simulink model "lab7"  (R2012b)
settings: Solver=ode45  StartTime=0.0  StopTime=720  RelTol=1e-3
undefined symbols (not defined in the file): des, gcbh
settings Model: Creator=gick  LastModifiedBy=gick

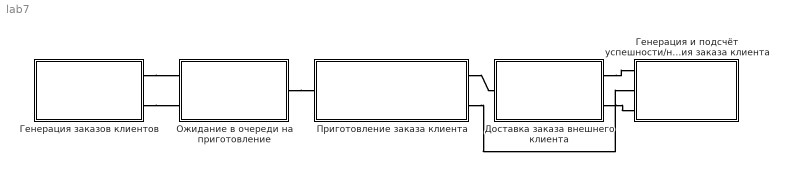
== system lab7 ==
  Генерация заказов клиентов : Subsystem
  Генерация и подсчёт успешности/неуспешности выполнения заказа клиента : Subsystem
  Доставка заказа внешнего клиента : Subsystem
  Ожидание в очереди на приготовление : Subsystem
  Приготовление заказа клиента : Subsystem
  connections:
  Генерация заказов клиентов/RConn1 -- Ожидание в очереди на приготовление/LConn1
  Генерация заказов клиентов/RConn2 -- Ожидание в очереди на приготовление/LConn2
  Ожидание в очереди на приготовление/RConn1 -- Приготовление заказа клиента/LConn1
  Приготовление заказа клиента/RConn1 -- Доставка заказа внешнего клиента/LConn1
  Приготовление заказа клиента/RConn2 -- Генерация и подсчёт успешности/неуспешности выполнения заказа клиента/LConn2
  Доставка заказа внешнего клиента/RConn1 -- Генерация и подсчёт успешности/неуспешности выполнения заказа клиента/LConn1
  Доставка заказа внешнего клиента/RConn2 -- Генерация и подсчёт успешности/неуспешности выполнения заказа клиента/LConn3

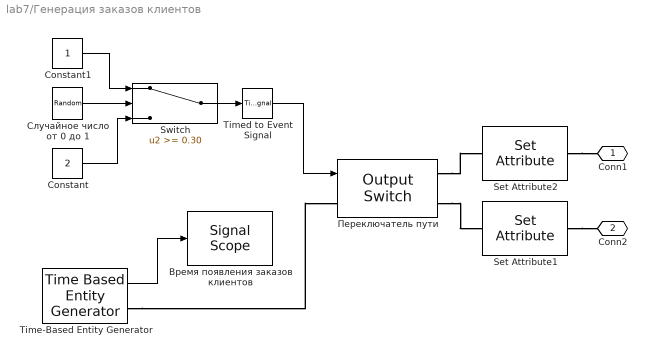
== system lab7/Генерация заказов клиентов ==
  Constant : Constant  Value=2
  Constant1 : Constant
  Set Attribute1 : SetAttribute  AttributeName=client_type  AttributeValue=2  EvaluatedAttributeValue={ 2 }
  Set Attribute2 : SetAttribute  AttributeName=client_type  EvaluatedAttributeValue={ 1 }
  Switch : Switch  Threshold=0.30
  Time-Based Entity Generator : TimeBasedEntityGenerator  Distribution=Exponential  InitialSeed=12  Mean=15  PriorityEntityGeneration=500  StatAverageIntergenerationTime=on
      settings: OutputPortMap=o2
  Timed to Event Signal : TimedToEventSignal
  Время появления заказов клиентов : SignalScope  LoadFcn=des.scope.CallbackSupport('seLoadFcn',gcbh)  StartFcn=des.scope.CallbackSupport('seStartFcn',gcbh)  StopFcn=des.scope.CallbackSupport('seStopFcn',gcbh)  ShowCountPlotted=on
      settings: CopyFcn=des.scope.CallbackSupport('seCopyFcn',gcbh)  DeleteFcn=des.scope.CallbackSupport('seDeleteFcn',gcbh)  PreSaveFcn=des.scope.CallbackSupport('sePreSaveFcn',gcbh)  NameChangeFcn=des.scope.CallbackSupport('seNameChangeFcn',gcbh)  OpenFcn=des.scope.CallbackSupport('seOpenFcn',gcbh)
  "Переключатель пути " : OutputSwitch  NumberOutputPorts=2  SwitchingCriterion=From signal port p
  Случайное число от 0 до 1 : UniformRandomNumber  Minimum=0  Seed=12  SampleTime=0.1
  Conn1 : PMIOPort  Port=1  Side=Right
  Conn2 : PMIOPort  Port=2  Side=Right
  wires:
  Случайное число от 0 до 1/1 -> Switch/2
  Switch/1 -> Timed to Event Signal/1
  Timed to Event Signal/1 -> "Переключатель пути "/1
  Time-Based Entity Generator/1 -> Время появления заказов клиентов/1
  Constant/1 -> Switch/3
  Constant1/1 -> Switch/1
  connections:
  Time-Based Entity Generator/RConn1 -- "Переключатель пути "/LConn1
  Set Attribute1/RConn1 -- Conn2/RConn1
  Set Attribute2/RConn1 -- Conn1/RConn1
  "Переключатель пути "/RConn1 -- Set Attribute2/LConn1
  "Переключатель пути "/RConn2 -- Set Attribute1/LConn1

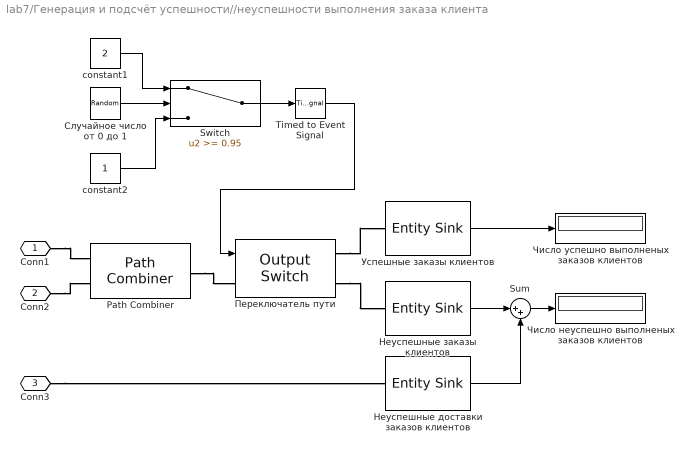
== system lab7/Генерация и подсчёт успешности//неуспешности выполнения заказа клиента ==
  Path Combiner : PathCombiner  NumberInputPorts=2
  Sum : Sum  Inputs=|++
  Switch : Switch  Threshold=0.95
  Timed to Event Signal : TimedToEventSignal
  constant1 : Constant  Value=2
  constant2 : Constant
  Неуспешные доставки заказов клиентов : EntitySink  StatNumberArrived=on
  Неуспешные заказы клиентов : EntitySink  StatNumberArrived=on
  "Переключатель пути " : OutputSwitch  NumberOutputPorts=2  SwitchingCriterion=From signal port p
  Случайное число от 0 до 1 : UniformRandomNumber  Minimum=0  Seed=12  SampleTime=0.1
  Успешные заказы клиентов : EntitySink  StatNumberArrived=on
  Число неуспешно выполненых заказов клиентов : Display
  Число успешно выполненых заказов клиентов : Display
  Conn1 : PMIOPort  Port=1  Side=Left
  Conn2 : PMIOPort  Port=2  Side=Left
  Conn3 : PMIOPort  Port=3  Side=Left
  wires:
  constant1/1 -> Switch/1
  constant2/1 -> Switch/3
  Случайное число от 0 до 1/1 -> Switch/2
  Switch/1 -> Timed to Event Signal/1
  Timed to Event Signal/1 -> "Переключатель пути "/1
  Успешные заказы клиентов/1 -> Число успешно выполненых заказов клиентов/1
  Неуспешные доставки заказов клиентов/1 -> Sum/2
  Неуспешные заказы клиентов/1 -> Sum/1
  Sum/1 -> Число неуспешно выполненых заказов клиентов/1
  connections:
  Path Combiner/RConn1 -- "Переключатель пути "/LConn1
  Conn1/RConn1 -- Path Combiner/LConn1
  Conn2/RConn1 -- Path Combiner/LConn2
  "Переключатель пути "/RConn1 -- Успешные заказы клиентов/LConn1
  "Переключатель пути "/RConn2 -- Неуспешные заказы клиентов/LConn1
  Conn3/RConn1 -- Неуспешные доставки заказов клиентов/LConn1

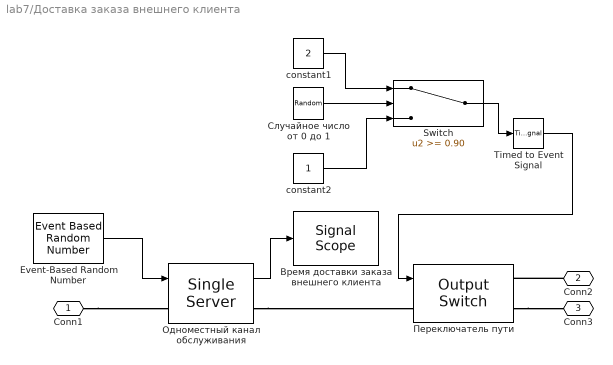
== system lab7/Доставка заказа внешнего клиента ==
  Event-Based Random Number : EventBasedRandomNumber  Distribution=Uniform  minUnif=10  maxUnif=50  Seed=12
  Switch : Switch  Threshold=0.90
  Timed to Event Signal : TimedToEventSignal
  constant1 : Constant  Value=2
  constant2 : Constant
  Время доставки заказа внешнего клиента : SignalScope  LoadFcn=des.scope.CallbackSupport('seLoadFcn',gcbh)  StartFcn=des.scope.CallbackSupport('seStartFcn',gcbh)  StopFcn=des.scope.CallbackSupport('seStopFcn',gcbh)  XMax=640  ShowCountPlotted=on
      settings: CopyFcn=des.scope.CallbackSupport('seCopyFcn',gcbh)  DeleteFcn=des.scope.CallbackSupport('seDeleteFcn',gcbh)  PreSaveFcn=des.scope.CallbackSupport('sePreSaveFcn',gcbh)  NameChangeFcn=des.scope.CallbackSupport('seNameChangeFcn',gcbh)  OpenFcn=des.scope.CallbackSupport('seOpenFcn',gcbh)  YMax=20
  Одноместный канал обслуживания : SingleServer  ServiceTimeFrom=Signal port t  AttributeName=ServTime  StatAverageWait=on
      settings: OutputPortMap=o4
  "Переключатель пути " : OutputSwitch  NumberOutputPorts=2  SwitchingCriterion=From signal port p
  Случайное число от 0 до 1 : UniformRandomNumber  Minimum=0  Seed=12  SampleTime=0.1
  Conn1 : PMIOPort  Port=1  Side=Left
  Conn2 : PMIOPort  Port=2  Side=Right
  Conn3 : PMIOPort  Port=3  Side=Right
  wires:
  Event-Based Random Number/1 -> Одноместный канал обслуживания/1
  Одноместный канал обслуживания/1 -> Время доставки заказа внешнего клиента/1
  constant1/1 -> Switch/1
  constant2/1 -> Switch/3
  Случайное число от 0 до 1/1 -> Switch/2
  Switch/1 -> Timed to Event Signal/1
  Timed to Event Signal/1 -> "Переключатель пути "/1
  connections:
  Conn1/RConn1 -- Одноместный канал обслуживания/LConn1
  Conn2/RConn1 -- "Переключатель пути "/RConn1
  Одноместный канал обслуживания/RConn1 -- "Переключатель пути "/LConn1
  "Переключатель пути "/RConn2 -- Conn3/RConn1

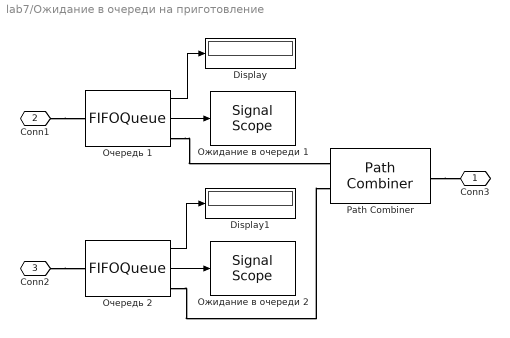
== system lab7/Ожидание в очереди на приготовление ==
  Display : Display
  Display1 : Display
  Path Combiner : PathCombiner  NumberInputPorts=2
  Ожидание в очереди 1 : SignalScope  LoadFcn=des.scope.CallbackSupport('seLoadFcn',gcbh)  StartFcn=des.scope.CallbackSupport('seStartFcn',gcbh)  StopFcn=des.scope.CallbackSupport('seStopFcn',gcbh)  ShowCountPlotted=on
      settings: CopyFcn=des.scope.CallbackSupport('seCopyFcn',gcbh)  DeleteFcn=des.scope.CallbackSupport('seDeleteFcn',gcbh)  PreSaveFcn=des.scope.CallbackSupport('sePreSaveFcn',gcbh)  NameChangeFcn=des.scope.CallbackSupport('seNameChangeFcn',gcbh)  OpenFcn=des.scope.CallbackSupport('seOpenFcn',gcbh)
  Ожидание в очереди 2 : SignalScope  LoadFcn=des.scope.CallbackSupport('seLoadFcn',gcbh)  StartFcn=des.scope.CallbackSupport('seStartFcn',gcbh)  StopFcn=des.scope.CallbackSupport('seStopFcn',gcbh)  ShowCountPlotted=on
      settings: CopyFcn=des.scope.CallbackSupport('seCopyFcn',gcbh)  DeleteFcn=des.scope.CallbackSupport('seDeleteFcn',gcbh)  PreSaveFcn=des.scope.CallbackSupport('sePreSaveFcn',gcbh)  NameChangeFcn=des.scope.CallbackSupport('seNameChangeFcn',gcbh)  OpenFcn=des.scope.CallbackSupport('seOpenFcn',gcbh)
  Очередь 1 : FIFOQueue  Capacity=10  StatNumberDeparted=on  StatAverageWait=on
      settings: OutputPortMap=o0,o2
  "Очередь 2 " : FIFOQueue  Capacity=10  StatNumberDeparted=on  StatAverageWait=on
      settings: OutputPortMap=o0,o2
  Conn3 : PMIOPort  Port=1  Side=Right
  Conn1 : PMIOPort  Port=2  Side=Left
  Conn2 : PMIOPort  Port=3  Side=Left
  wires:
  Очередь 1/2 -> Ожидание в очереди 1/1
  "Очередь 2 "/2 -> Ожидание в очереди 2/1
  Очередь 1/1 -> Display/1
  "Очередь 2 "/1 -> Display1/1
  connections:
  "Очередь 2 "/RConn1 -- Path Combiner/LConn2
  Path Combiner/RConn1 -- Conn3/RConn1
  Очередь 1/RConn1 -- Path Combiner/LConn1
  Conn1/RConn1 -- Очередь 1/LConn1
  Conn2/RConn1 -- "Очередь 2 "/LConn1

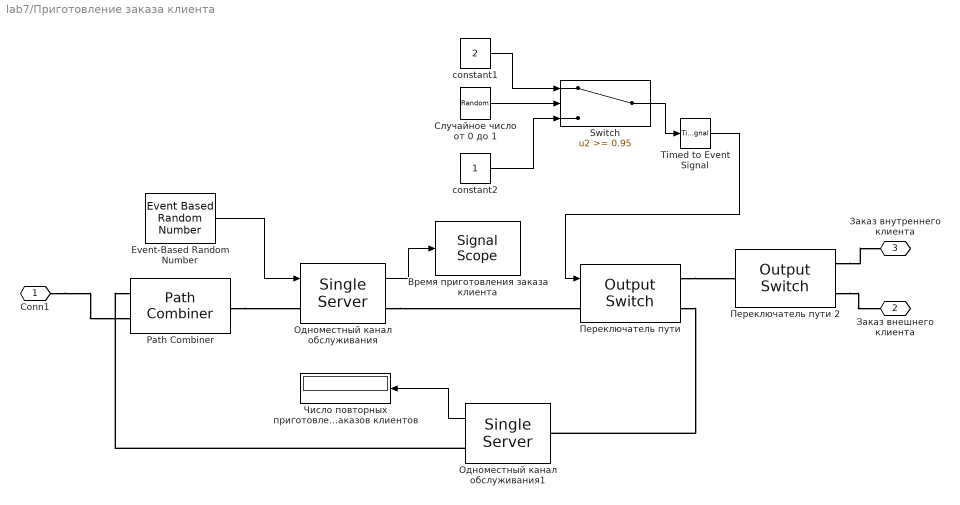
== system lab7/Приготовление заказа клиента ==
  Event-Based Random Number : EventBasedRandomNumber  Distribution=Uniform  minUnif=5  maxUnif=20  Seed=12
  Path Combiner : PathCombiner  NumberInputPorts=2
  Switch : Switch  Threshold=0.95
  Timed to Event Signal : TimedToEventSignal
  constant1 : Constant  Value=2
  constant2 : Constant
  Время приготовления заказа клиента : SignalScope  LoadFcn=des.scope.CallbackSupport('seLoadFcn',gcbh)  StartFcn=des.scope.CallbackSupport('seStartFcn',gcbh)  StopFcn=des.scope.CallbackSupport('seStopFcn',gcbh)  XMax=640  ShowCountPlotted=on
      settings: CopyFcn=des.scope.CallbackSupport('seCopyFcn',gcbh)  DeleteFcn=des.scope.CallbackSupport('seDeleteFcn',gcbh)  PreSaveFcn=des.scope.CallbackSupport('sePreSaveFcn',gcbh)  NameChangeFcn=des.scope.CallbackSupport('seNameChangeFcn',gcbh)  OpenFcn=des.scope.CallbackSupport('seOpenFcn',gcbh)  YMax=20
  Одноместный канал обслуживания : SingleServer  ServiceTimeFrom=Signal port t  AttributeName=ServTime  StatAverageWait=on
      settings: OutputPortMap=o4
  Одноместный канал обслуживания1 : SingleServer  AttributeName=ServTime  StatNumberDeparted=on
  "Переключатель пути " : OutputSwitch  NumberOutputPorts=2  SwitchingCriterion=From signal port p
  Переключатель пути 2 : OutputSwitch  NumberOutputPorts=2  SwitchingCriterion=From attribute  AttributeName=client_type
  Случайное число от 0 до 1 : UniformRandomNumber  Minimum=0  Seed=12  SampleTime=0.1
  Число повторных приготовлений заказов клиентов : Display
  Conn1 : PMIOPort  Port=1  Side=Left
  Заказ внешнего клиента : PMIOPort  Port=2  Side=Right
  Заказ внутреннего клиента : PMIOPort  Port=3  Side=Right
  wires:
  constant1/1 -> Switch/1
  constant2/1 -> Switch/3
  Случайное число от 0 до 1/1 -> Switch/2
  Switch/1 -> Timed to Event Signal/1
  Timed to Event Signal/1 -> "Переключатель пути "/1
  Одноместный канал обслуживания/1 -> Время приготовления заказа клиента/1
  Event-Based Random Number/1 -> Одноместный канал обслуживания/1
  Одноместный канал обслуживания1/1 -> Число повторных приготовлений заказов клиентов/1
  connections:
  Одноместный канал обслуживания/RConn1 -- "Переключатель пути "/LConn1
  Conn1/RConn1 -- Path Combiner/LConn2
  Path Combiner/RConn1 -- Одноместный канал обслуживания/LConn1
  "Переключатель пути "/RConn1 -- Переключатель пути 2/LConn1
  Переключатель пути 2/RConn1 -- Заказ внутреннего клиента/RConn1
  Переключатель пути 2/RConn2 -- Заказ внешнего клиента/RConn1
  "Переключатель пути "/RConn2 -- Одноместный канал обслуживания1/LConn1
  Одноместный канал обслуживания1/RConn1 -- Path Combiner/LConn1
